simulink model "Record_and_view_L1_Signal"  (R2018b)
settings: Solver=VariableStepAuto  StartTime=0.0  StopTime=90  RelTol=1e-3
libraries: dspswit3 x1, sdrrlib x1, rtlsdr_book_library x1
settings Model: Creator=Smalls  LastModifiedBy=paulb
settings DebuggingCC: LibraryContextMissingDiagnostic=none
settings SFSimCC: SimUseLocalCustomCode=off
settings RTWCC: RTWUseLocalCustomCode=off

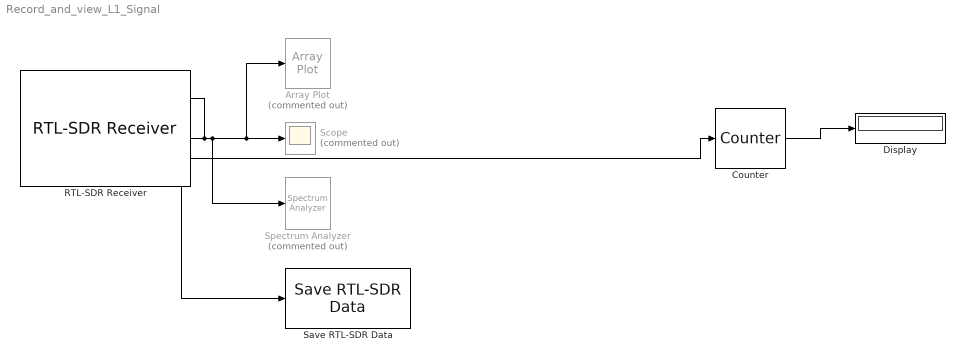
== system Record_and_view_L1_Signal ==
  Array Plot : ArrayPlot  Commented=on
  Counter : dspswit3/Counter  Direction=Up  CountEvent=Non-zero sample  CounterSize=32 bits  MaxCount=255  InitialCount=0  Output=Count  HitValue=32  ResetInput=off  SamplesPerFrame=1  Ts=1  CntDtype=double  HitDtype=Logical
  Display : Display
  RTL-SDR Receiver : sdrrlib/RTL-SDR Receiver  IPAddress=0  CenterFrequencySource=Dialog  CenterFrequency=1575.32e6  GainSource=AGC  Gain=100  ADCRate=1.5e6  FrequencyCorrection=0  LostSamplesOutputPort=on  LatencyOutputPort=off  OutputDataType=int16  FrameLength=1024  EnableBurstMode=off  NumFramesInBurst=20  sobjType=sdrr.internal.SDRRTLReceiverSL  dataUDPPort=-1  ctrlUDPPort=-1  subDeviceList=nosubdev  sdrBlockType=SDRBlockTypeSLT.SDRRxBlock  requester=UNUSED_BY_SFCN  sdrExecutionMode=SDRExecutionModeSLT.ExecModeHW  BypassUserLogic=off  DecimatorSelect=DDC decimator  SourceSelect=RF data  SineAmplitude=16000  EnableInternalClock=off  BypassIQBalance=off  IFBandwidth=40e6  ADCRateSource=Dialog  IntermediateFrequency=0  DecimationFactorSource=Dialog  DecimationFactor=512  RFFrequencyIsTunable=logical(0)  SampleTime=(1024)/(1.5e6)  IFBandwidthSource=Dialog  SineFrequency=30000  BypassDCBlockingFilter=off  IntermediateFrequencySource=Dialog  IQBalanceCoefficients=64  SkipAllHardwareResetAndInitialization=off  EnableIQCalibrationTable=on  CacheIQCalibrationTable=off  EnableOffsetTuning=off  EnableRTLAGC=off  EnableTestMode=off  EnableTunerAGC=on  FrequencyCorrectionSource=Dialog  NumMLBuffers=128  NumUSBBuffers=16  RTLCrystalFrequency=28800000  TunerCrystalFrequency=28800000
      settings: SourceProductName=Communications System Toolbox Support Package for RTL-SDR Radio  SourceProductBaseCode=RTLSDR
  Save RTL-SDR Data : rtlsdr_book_library/Additional Tools/Save RTL-SDR Data  file_name=C:\sandbox\SW RX demo\datalogs\test_1p5MHz_1kHz_figure8_5.mat
      settings: SourceProductName=RTL-SDR Book Library
  Scope : Scope  Commented=on
  Spectrum Analyzer : SpectrumAnalyzer  Commented=on
  wires:
  RTL-SDR Receiver/1 -> Save RTL-SDR Data/1, Spectrum Analyzer/1, Array Plot/1, Scope/1
  RTL-SDR Receiver/2 -> Counter/1
  Counter/1 -> Display/1
